simulink model "at_slk_Sensor2Phy"  (R2017b)
settings: Solver=FixedStepDiscrete  StartTime=0.0  StopTime=10.0  FixedStep=1  RelTol=1e-3
PreLoadFcn:
  | sl_refresh_customizations
  | simulinkExportUnitCs
  | E_Global_Constants
  | A_Data_Dictionary
  | 
  | 
  | 
  | 
  | 
  | enum_Simulink
  | 
  | bus_Simulink
InitFcn:
  | checkUnitMismatch
model workspace (MAT data in the model file):
  ESD_URL = 'http://127.0.0.1:63320/node?ref=r%3A92f02917-2939-4625-878a-0cf4bf3cdc0b%28AHCDemo._30_Implementation%29%2F6499409138675363509'
settings Model: Creator=ohm9xd  LastModifiedBy=oezqk7
settings OptimizationCC: DefaultParameterBehavior=Inlined  PassReuseOutputArgsAs=Individual arguments  ZeroExternalMemoryAtStartup=off
settings DebuggingCC: SignalRangeChecking=error  InheritedTsInSrcMsg=none  ParameterTunabilityLossMsg=error
settings SFSimCC: MATLABDynamicMemAlloc=off
settings RTWCC: SystemTargetFile=esd_ert.tlc  GenCodeOnly=on  TemplateMakefile=ert_default_tmf  Description=CSD  GenerateReport=on  IncludeHyperlinkInReport=on  LaunchReport=on  GenerateTraceInfo=on  GenerateTraceReport=on  GenerateTraceReportSl=on  GenerateTraceReportSf=on  GenerateTraceReportEml=on
settings CodeAppCC: ForceParamTrailComments=on  IgnoreCustomStorageClasses=off  OperatorAnnotations=on  SimulinkDataObjDesc=on  SFDataObjDesc=on  InsertBlockDesc=on
settings STFCustomTargetCC: TargetLangStandard=C99 (ISO)  MultiwordLength=256  GenerateSampleERTMain=on  IncludeMdlTerminateFcn=off  CombineOutputUpdateFcns=on  CombineSignalStateStructs=on  SuppressErrorStatus=on  ERTCustomFileBanners=on  MultiInstanceERTCode=on  CodeInterfacePackaging=Reusable function  SupportContinuousTime=off  SupportNonInlinedSFcns=off  RemoveDisableFunc=on  RemoveResetFunc=on  MATLABClassNameForMDSCustomization=Simulink.SoftwareTarget.ERTCustomization  GRTInterface=off  SystemTargetFile=esd_ert.tlc
settings ERTTargetCC: TargetLangStandard=C99 (ISO)  GenerateSampleERTMain=on  ParMdlRefBuildCompliant=off  CompOptLevelCompliant=off  ConcurrentExecutionCompliant=off  IncludeMdlTerminateFcn=off  CombineSignalStateStructs=on  SuppressErrorStatus=on  MultiInstanceERTCode=on  CodeInterfacePackaging=Reusable function  RemoveDisableFunc=on  ModelStepFunctionPrototypeControlCompliant=off  CPPClassGenCompliant=off  UseToolchainInfoCompliant=off  InlinedParameterPlacement=NonHierarchical  ERTCustomFileTemplate=example_file_process.tlc

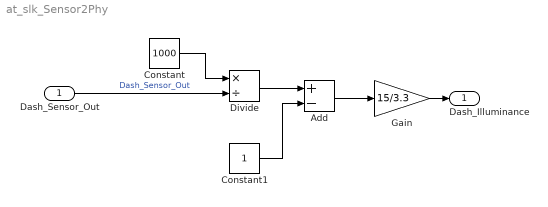
== system at_slk_Sensor2Phy ==
  Dash_Sensor_Out : Inport  OutDataTypeStr=double  Unit=V
      settings: AttributesFormatString=(V)
  Add : Sum  Inputs=+-
  Constant : Constant  Value=1000
  Constant1 : Constant
  Divide : Product  Inputs=*/
  Gain : Gain  Gain=15/3.3
  Dash_Illuminance : Outport  OutDataTypeStr=double  Unit=lx
      settings: AttributesFormatString=(lx)
  wires:
  Dash_Sensor_Out/1 -> Divide/2  "Dash_Sensor_Out"
  Gain/1 -> Dash_Illuminance/1
  Constant/1 -> Divide/1
  Divide/1 -> Add/1
  Constant1/1 -> Add/2
  Add/1 -> Gain/1
